simulink model "sampling_bandpass_lab_experiment2"  (R2020b)
settings: Solver=ode45  StartTime=0.0  StopTime=2*0.002097  RelTol=1e-3  EnableMultiTasking=on
libraries: dsparch4 x1
settings Model: Creator=morelos_zaragoza  LastModifiedBy=14083
settings DataIOCC: LimitDataPoints=on  SaveFormat=Array  SignalLoggingSaveFormat=ModelDataLogs  ReturnWorkspaceOutputs=off
settings OptimizationCC: ExpressionDepthLimit=2147483647  InitFltsAndDblsToZero=on  LifeSpan=inf
settings DebuggingCC: SaveWithParameterizedLinksMsg=none  UnderspecifiedInitializationDetection=Classic  MergeDetectMultiDrivingBlocksExec=none  SignalResolutionControl=TryResolveAllWithWarning  SolverPrmCheckMsg=warning  MultiTaskDSMMsg=warning  MultiTaskCondExecSysMsg=none  FcnCallInpInsideContextMsg=warning  StateNameClashWarn=warning  SFUnexpectedBacktrackingDiag=warning  SFNoUnconditionalDefaultTransitionDiag=warning  SFExecutionAtInitializationDiag=none  ArithmeticOperatorsInVariantConditions=warning
settings HardwareCC: ProdBitPerPointer=32  ProdBitPerSizeT=32  ProdBitPerPtrDiffT=32  ProdLargestAtomicFloat=None  ProdIntDivRoundTo=Undefined  ProdEndianess=Unspecified  ProdWordSize=32  ProdHWDeviceType=32-bit Generic
settings ModelReferenceCC: PropagateSignalLabelsOutOfModel=off
settings SFSimCC: SimUseLocalCustomCode=off  CustomCodeUndefinedFunction=UseInterfaceOnly
settings RTWCC: RTWUseLocalCustomCode=off
settings CodeAppCC: StateflowObjectComments=on
settings GRTTargetCC: TargetFcnLib=ansi_tfl_tmw.mat  TargetLangStandard=C89/C90 (ANSI)  CombineOutputUpdateFcns=off  GRTInterface=on
settings ConfigComp: CovMetricSettings=dw  CovSaveCumulativeToWorkspaceVar=on  CovSaveSingleToWorkspaceVar=on  CovExternalEMLEnable=off

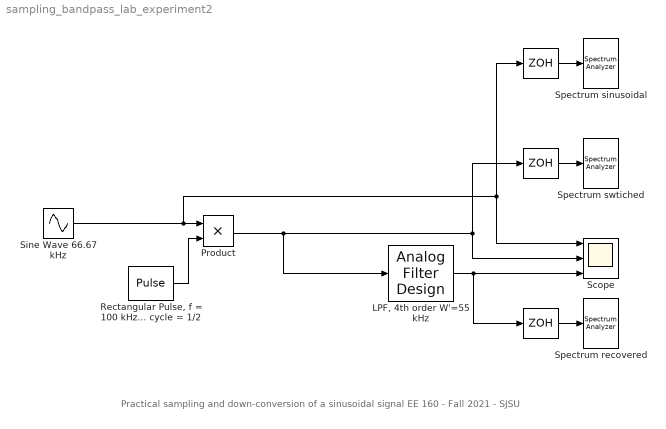
== system sampling_bandpass_lab_experiment2 ==
  note: Practical sampling and down-conversion of a sinusoidal signal
      | EE 160 - Fall 2021 - SJSU
  " " : ZeroOrderHold  SampleTime=1/200000
  "  " : ZeroOrderHold  SampleTime=1/200000
  "   " : ZeroOrderHold  SampleTime=1/200000
  "LPF, 4th order W'=55 kHz" : dsparch4/Analog Filter Design  method=Butterworth  filttype=Lowpass  N=4  Wlo=2*pi*55000  Whi=2*pi*110  Rp=2  Rs=40
  Product : Product  RndMeth=Zero
  "Rectangular Pulse, f = 100 kHz Dute cycle = 1/2" : DiscretePulseGenerator  PulseType=Time based  Period=1/100000  PulseWidth=50  SampleTime=1e-2/2)
  Scope : Scope  NumInputPorts=3
  Sine Wave 66.67 kHz : Sin  Frequency=2*pi*66670  SampleTime=1/66670000
  Spectrum recovered : SpectrumAnalyzer
  Spectrum sinusoidal : SpectrumAnalyzer
  Spectrum swtiched : SpectrumAnalyzer
  wires:
  "Rectangular Pulse, f = 100 kHz Dute cycle = 1/2"/1 -> Product/2
  Product/1 -> "  "/1, Scope/2, "LPF, 4th order W'=55 kHz"/1
  "  "/1 -> Spectrum swtiched/1
  Sine Wave 66.67 kHz/1 -> Product/1, Scope/1, "   "/1
  "LPF, 4th order W'=55 kHz"/1 -> Scope/3, " "/1
  " "/1 -> Spectrum recovered/1
  "   "/1 -> Spectrum sinusoidal/1
